simulink model "Regen_block"  (R2024b)
settings: Solver=VariableStepAuto  StartTime=0.0  StopTime=10.0  RelTol=1e-3
model workspace (MAT data in the model file):
  Actual_Brake_bias = 4
  Actual_brake_bias = 1.5
undefined symbols (not defined in the file or in its folder): A1, ended, GND, Single
libraries: canmsglib x2, raspberrypiBasiclib x1, raspberrypiCommlib x1
settings Model: Creator=shrav  LastModifiedBy=shrav

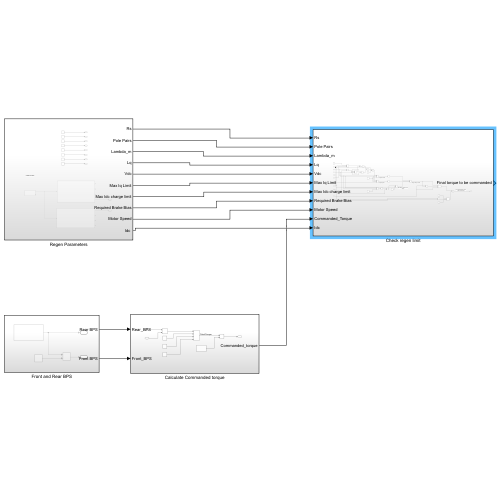
[thumbnail: Simulink's stored preview of the top-level diagram]
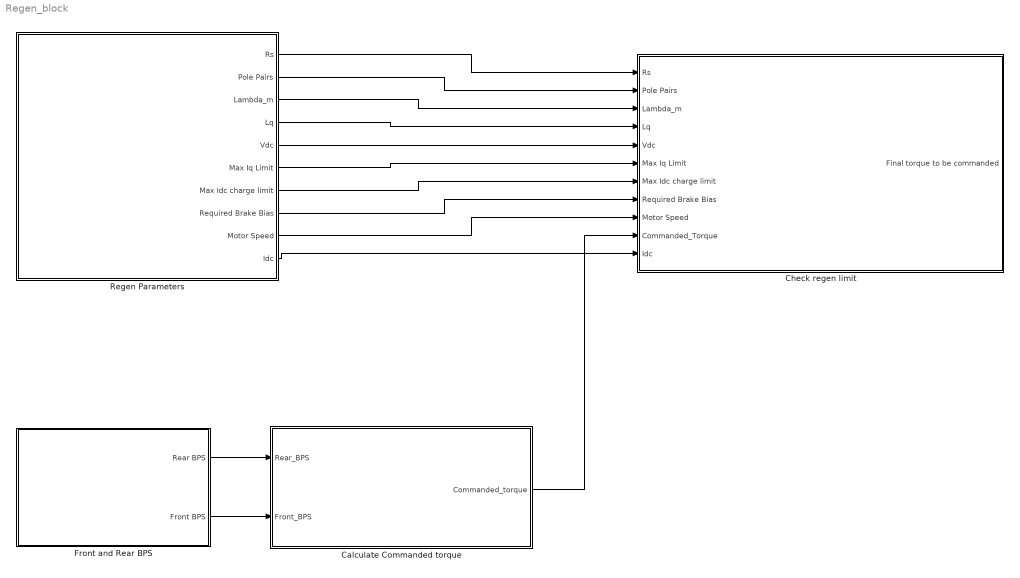
== system Regen_block ==
  Calculate Commanded torque : Subsystem
  Check regen limit : Subsystem
  Front and Rear BPS : Subsystem
  Regen Parameters : Subsystem
  wires:
  Front and Rear BPS/1(Rear BPS) -> Calculate Commanded torque/1(Rear_BPS)
  Front and Rear BPS/2(Front BPS) -> Calculate Commanded torque/2(Front_BPS)
  Regen Parameters/1(Rs) -> Check regen limit/1(Rs)
  Regen Parameters/2(Pole Pairs) -> Check regen limit/2(Pole Pairs)
  Regen Parameters/3(Lambda_m) -> Check regen limit/3(Lambda_m)
  Regen Parameters/4(Lq) -> Check regen limit/4(Lq)
  Regen Parameters/5(Vdc) -> Check regen limit/5(Vdc)
  Regen Parameters/6(Max Iq Limit) -> Check regen limit/6(Max Iq Limit)
  Regen Parameters/7(Max Idc charge limit) -> Check regen limit/7(Max Idc charge limit)
  Regen Parameters/8(Required Brake Bias) -> Check regen limit/8(Required Brake Bias)
  Regen Parameters/9(Motor Speed) -> Check regen limit/9(Motor Speed)
  Calculate Commanded torque/1(Commanded_torque) -> Check regen limit/10(Commanded_Torque)
  Regen Parameters/10("Idc ") -> Check regen limit/11(Idc)

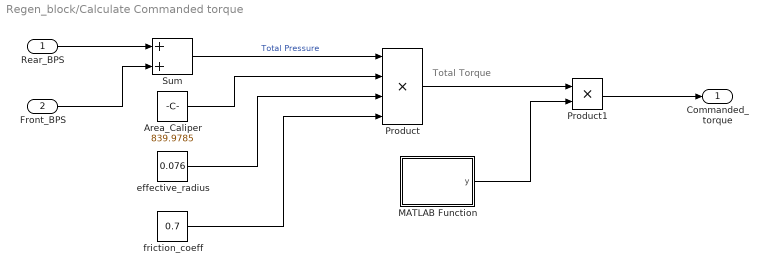
== system Regen_block/Calculate Commanded torque ==
  note: Total Torque
  Rear_BPS : Inport
  Front_BPS : Inport  Port=2
  Area_Caliper : Constant  Value=839.9785
  MATLAB Function : MATLAB Function  TreatAsAtomicUnit=on
  Product : Product  Inputs=4
  Product1 : Product
  Sum : Sum
  effective_radius : Constant  Value=0.076
  friction_coeff : Constant  Value=0.7
  Commanded_torque : Outport
  wires:
  Rear_BPS/1 -> Sum/1
  Front_BPS/1 -> Sum/2
  Sum/1 -> Product/1  "Total Pressure"
  Area_Caliper/1 -> Product/2
  effective_radius/1 -> Product/3
  friction_coeff/1 -> Product/4
  Product/1 -> Product1/1
  Product1/1 -> Commanded_torque/1
  MATLAB Function/1(y) -> Product1/2

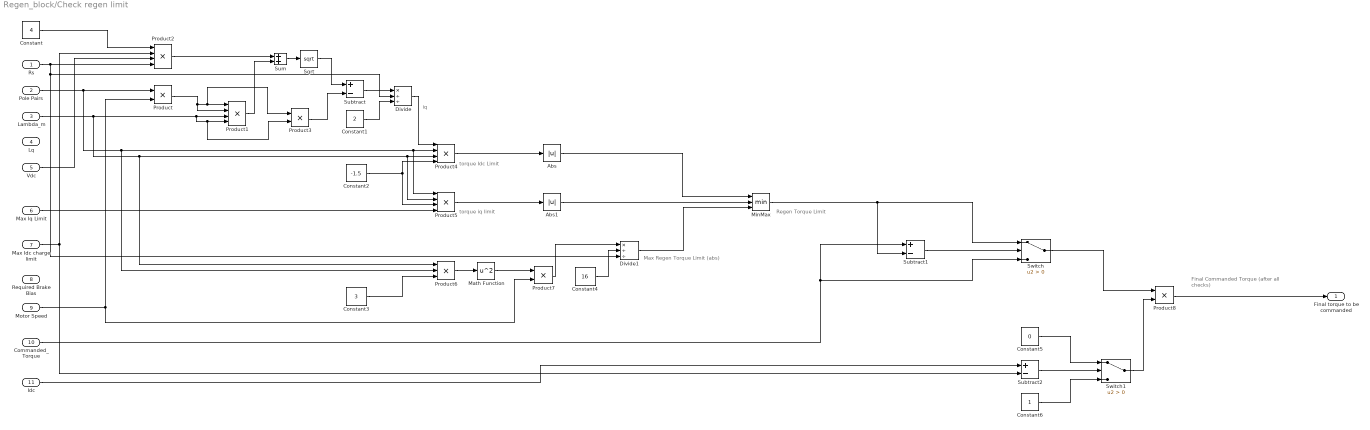
== system Regen_block/Check regen limit ==
  note: Final Commanded Torque
      | (after all checks)
  note: Regen Torque Limit
  note: Max Regen Torque Limit
      | (abs)
  note: torque iq limit
  note: torque Idc Limit
  note: iq
  Rs : Inport
  Pole Pairs : Inport  Port=2
  Lambda_m : Inport  Port=3
  Lq : Inport  Port=4
  Vdc : Inport  Port=5
  Max Iq Limit : Inport  Port=6
  Max Idc charge limit : Inport  Port=7
  Required Brake Bias : Inport  Port=8
  Motor Speed : Inport  Port=9
  Commanded_Torque : Inport  Port=10
  Idc : Inport  Port=11
  Abs : Abs  SaturateOnIntegerOverflow=off
  Abs1 : Abs  SaturateOnIntegerOverflow=off
  Constant : Constant  Value=4
  Constant1 : Constant  Value=2
  Constant2 : Constant  Value=-1.5
  Constant3 : Constant  Value=3
  Constant4 : Constant  Value=16
  Constant5 : Constant  Value=0
  Constant6 : Constant
  Divide : Product  Inputs=*//
  Divide1 : Product  Inputs=*//
  Math Function : Math  Operator=square
  MinMax : MinMax  Inputs=3
  Product{,3,7..8} (4 alike) : Product
  Product{1..2,4..5} (4 alike) : Product  Inputs=4
  Product6 : Product  Inputs=3
  Sqrt : Sqrt
  Subtract : Sum  Inputs=+-
  Subtract1 : Sum  Inputs=+-
  Subtract2 : Sum  Inputs=+-
  Sum : Sum
  Switch : Switch  Criteria=u2 > Threshold  SaturateOnIntegerOverflow=off  InputSameDT=off
  Switch1 : Switch  Criteria=u2 > Threshold  SaturateOnIntegerOverflow=off  InputSameDT=off
  Final torque to be commanded : Outport
  wires:
  Pole Pairs/1 -> Product6/2, Product5/1, Product4/2, Product/1
  Motor Speed/1 -> Product7/2, Product/2
  Product/1 -> Product1/2, Product3/1, Product1/1
  Lambda_m/1 -> Product6/1, Product5/2, Product4/3, Product3/2, Product1/4, Product1/3
  Rs/1 -> Divide1/3, Divide/2, Product2/4
  Vdc/1 -> Product2/3
  Max Idc charge limit/1 -> Subtract2/2, Product2/2
  Constant/1 -> Product2/1
  Product2/1 -> Sum/1
  Product1/1 -> Sum/2
  Sum/1 -> Sqrt/1
  Sqrt/1 -> Subtract/1
  Product3/1 -> Subtract/2
  Subtract/1 -> Divide/1
  Constant1/1 -> Divide/3
  Divide/1 -> Product4/1
  Constant2/1 -> Product5/3, Product4/4
  Product4/1 -> Abs/1
  Max Iq Limit/1 -> Product5/4
  Product5/1 -> Abs1/1
  Constant3/1 -> Product6/3
  Product6/1 -> Math Function/1
  Math Function/1 -> Product7/1
  Product7/1 -> Divide1/1
  Constant4/1 -> Divide1/2
  Divide1/1 -> MinMax/3
  Abs1/1 -> MinMax/2
  Abs/1 -> MinMax/1
  Commanded_Torque/1 -> Switch/3, Subtract1/1
  MinMax/1 -> Switch/1, Subtract1/2
  Subtract1/1 -> Switch/2
  Idc/1 -> Subtract2/1
  Subtract2/1 -> Switch1/2
  Constant5/1 -> Switch1/1
  Constant6/1 -> Switch1/3
  Switch/1 -> Product8/1
  Switch1/1 -> Product8/2
  Product8/1 -> Final torque to be commanded/1

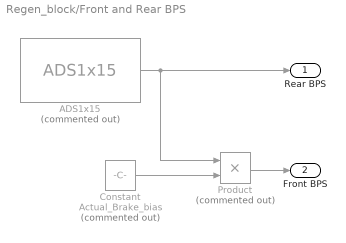
== system Regen_block/Front and Rear BPS ==
  ADS1x15 : raspberrypiBasiclib/ADS1x15  Commented=on  ADCChip=ADS1015  I2CAddress=0x48  ConversionMode=Single-shot  InputConfiguration=A1 - GND (Single-ended)  GainConfigurationDifferential=+/- 2.048 V  GainConfigurationSingleEnded=1.024 V  DataRateConfigurationADS1015=3300SPS  DataRateConfigurationADS1115=128SPS  SampleTime=0.01  EnableComparatorMode=off  ComparatorMode=Traditional with hysterisis  ComparatorPolarityConfiguration=Active low  ComparatorLatchingConfiguration=Non-latching  ComparatorQueueConfiguration=Assert after 1 conversion  ComparatorLowThresholdADS1015=0  ComparatorLowThresholdADS1115=0  ComparatorHighThresholdADS1015=0  ComparatorHighThresholdADS1115=0
  Constant : Constant  Commented=on  Value=Actual_Brake_bias
  Product : Product  Commented=on
  Rear BPS : Outport
  Front BPS : Outport  Port=2
  wires:
  ADS1x15/1 -> Product/1, Rear BPS/1
  Product/1 -> Front BPS/1
  Constant/1 -> Product/2

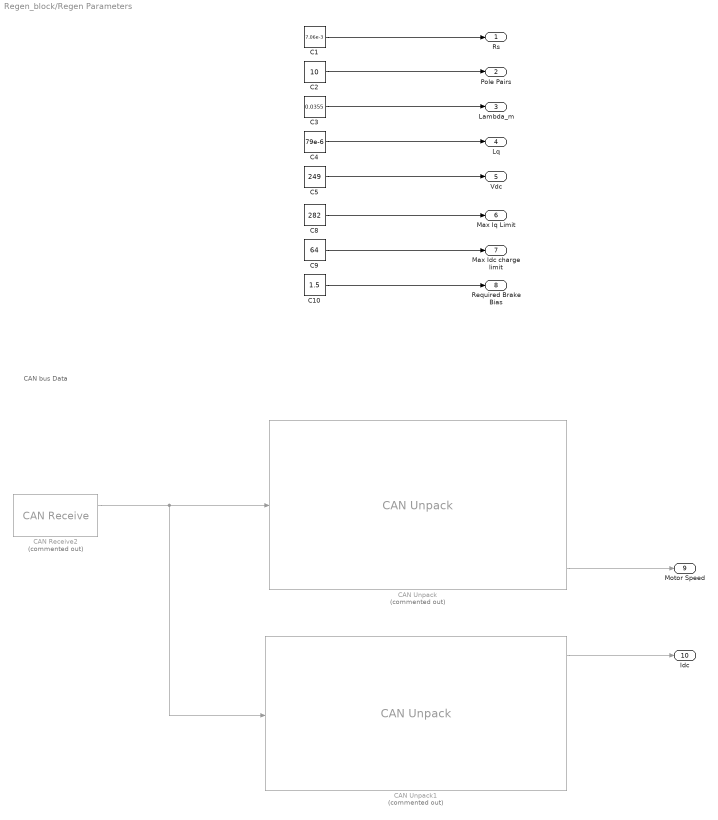
== system Regen_block/Regen Parameters ==
  note: CAN bus Data
  C1 : Constant  Value=7.06e-3
  C10 : Constant  Value=1.5
  C2 : Constant  Value=10
  C3 : Constant  Value=0.0355
  C4 : Constant  Value=79e-6
  C5 : Constant  Value=249
  C8 : Constant  Value=282
  C9 : Constant  Value=64
  CAN Receive2 : raspberrypiCommlib/CAN Receive  Commented=on  DeviceID=can0  SetupCAN=off  TypeofCAN=Real  OutputDataType=CAN Msg  IdentifierType=Standard (11-bit identifier)  MessageId=100  MsgLength=8  SampleTime=-1  OutputError=off  OutputRemote=off  SimulateUsing=Code generation
  CAN Unpack : canmsglib/CAN Unpack  Commented=on  CANdbFile=C:\Users\shrav\Downloads\rfr25can0.dbc  MsgList=M165_Motor_Position_Info  MsgName=M165_Motor_Position_Info  MsgIDType=Standard (11-bit identifier)  MsgIdentifier=165  MsgLength=8  SignalInfo={'INV_Delta_Resolver_Filtered','48','16','LE','signed','Standard','0','0.1','0','-3276.8','3276.7';'INV_Electrical_Output_Frequency','32','16','LE','signed','Standard','0','0.1','0','-3276.8','3276.7';'INV_Motor_Angle_Electrical','0','16','LE','unsigned','Standard','0','0.1','0','0','6553.5';'INV_Motor_Speed','16','16','LE','signed','Standard','0','1','0','-32768','32767'}  IDPort=off  TimestampPort=off  ErrorPort=off  RemotePort=off  LengthPort=off  StatusPort=off  ApplyMinMax=off
      settings: DataFormat=CANdb specified signals
  CAN Unpack1 : canmsglib/CAN Unpack  Commented=on  CANdbFile=C:\Users\shrav\Downloads\rfr25can0.dbc  MsgList=M166_Current_Info  MsgName=M166_Current_Info  MsgIDType=Standard (11-bit identifier)  MsgIdentifier=166  MsgLength=8  SignalInfo={'INV_DC_Bus_Current','48','16','LE','signed','Standard','0','0.1','0','-3276.8','3276.7';'INV_Phase_A_Current','0','16','LE','signed','Standard','0','0.1','0','-3276.8','3276.7';'INV_Phase_B_Current','16','16','LE','signed','Standard','0','0.1','0','-3276.8','3276.7';'INV_Phase_C_Current','32','16','LE','signed','Standard','0','0.1','0','-3276.8','3276.7'}  IDPort=off  TimestampPort=off  ErrorPort=off  RemotePort=off  LengthPort=off  StatusPort=off  ApplyMinMax=off
      settings: LibrarySourceBlock=canlib/CAN Unpack  DataFormat=CANdb specified signals
  Rs : Outport
  Pole Pairs : Outport  Port=2
  Lambda_m : Outport  Port=3
  Lq : Outport  Port=4
  Vdc : Outport  Port=5
  Max Iq Limit : Outport  Port=6
  Max Idc charge limit : Outport  Port=7
  Required Brake Bias : Outport  Port=8
  Motor Speed : Outport  Port=9
  "Idc " : Outport  Port=10
  wires:
  C1/1 -> Rs/1
  C2/1 -> Pole Pairs/1
  C3/1 -> Lambda_m/1
  C4/1 -> Lq/1
  C5/1 -> Vdc/1
  C8/1 -> Max Iq Limit/1
  C9/1 -> Max Idc charge limit/1
  C10/1 -> Required Brake Bias/1
  CAN Unpack/4 -> Motor Speed/1
  CAN Receive2/1 -> CAN Unpack1/1, CAN Unpack/1
  CAN Unpack1/1 -> "Idc "/1

== matlab function Regen_block/Calculate Commanded torque/MATLAB Function ==
  data: y output
function y = fcn()

a = 0.8;  % if initial brake bias is 80:20 , then a is 0.8

b = 1.5;  % this is required brake bias ( 60:40 ) .
y = ((a/b)+(a-1));
